simulink model "hpt_frt_model"  (R2025a)
settings: Solver=ode3  StartTime=0.0  StopTime=0.5  FixedStep=1e-05  RelTol=1e-3
undefined symbols (not defined in the file or in its folder): D1, Delta
libraries: spsSeriesRLCBranchLib x5, spsUniversalBridgeLib x4, spsLinearTransformerLib x3, spsThreePhaseFaultLib x2, spsThreePhaseVIMeasurementLib x2, spsBreakerLib x1, spsThreePhaseSourceLib x1, spsThreePhaseParallelRLCLoadLib x1, spsThreePhaseTransformerTwoWindingsLib x1, spsVoltageMeasurementLib x1, sps_lib x1
settings Model: Creator=m1391  LastModifiedBy=m1391

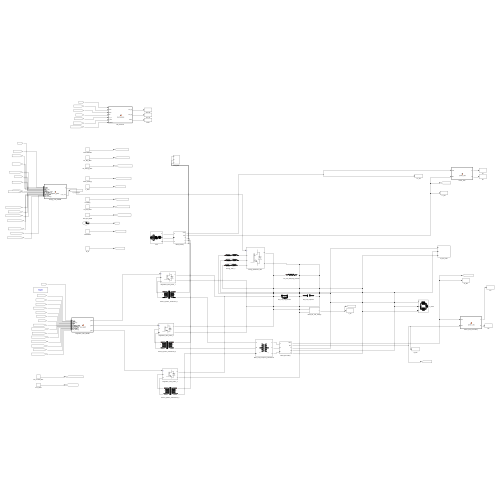
[thumbnail: Simulink's stored preview of the top-level diagram]
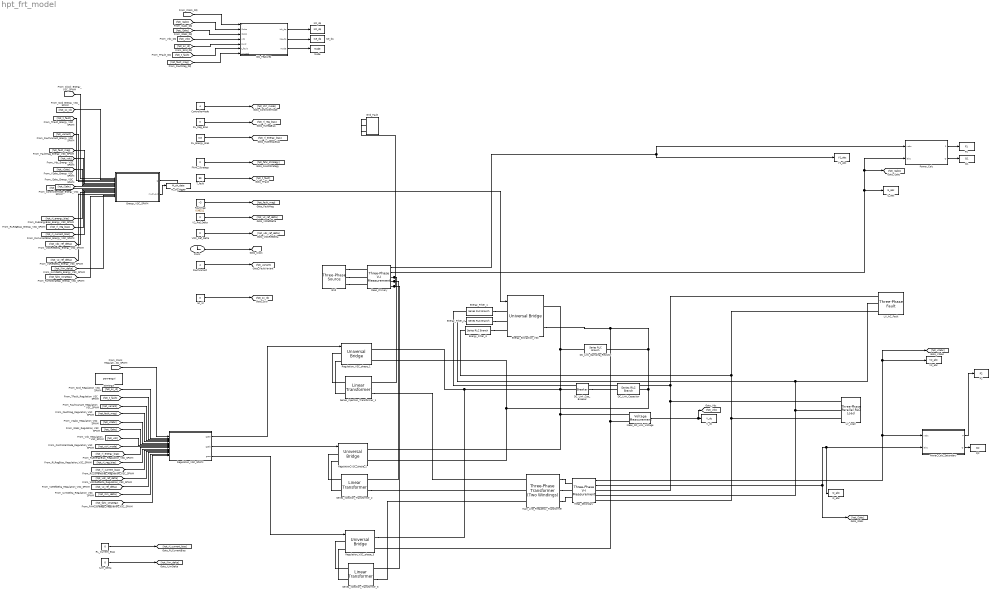
== system hpt_frt_model ==
  Clock : Clock
  ControllerMode : Constant  Value=4
  DC_Link_Cap_Breaker : spsBreakerLib/Breaker  InitialState=1  SwitchingTimes=[99]  External=off  BreakerResistance=0.01  SnubberResistance=1e6  SnubberCapacitance=inf  Measurements=None  MoreParameters=on  NoBreakLoop=off
  DC_Link_Capacitor : spsSeriesRLCBranchLib/Series RLC Branch  LConnTagsString=__new0  RConnTagsString=__new0  BranchType=C  Resistance=1  Inductance=1e-3  SetiL0=off  InitialCurrent=0  Capacitance=2200e-6  Setx0=on  InitialVoltage=800  Measurements=None
  DC_Link_Damping_Resistor : spsSeriesRLCBranchLib/Series RLC Branch  LConnTagsString=__new0  RConnTagsString=__new0  BranchType=R  Resistance=8.2  Inductance=1e-3  SetiL0=off  InitialCurrent=0  Capacitance=1e-6  Setx0=off  InitialVoltage=0  Measurements=None
  DQ_Features : MATLAB Function  TreatAsAtomicUnit=on
  Energy_Extraction_VSC : spsUniversalBridgeLib/Universal Bridge  Arms=3  SnubberResistance=1e5  SnubberCapacitance=1e-9  Device=IGBT / Diodes  Ron=1e-3  Lon=0  ForwardVoltages="[  0  0  ]"  ForwardVoltage=0  GTOparameters=[ 10e-6 , 20e-6 ]  IGBTparameters=[ 1e-6 , 2e-6 ]  Measurements=All voltages and currents  Measurements_2=None  converterType=Rectifier
  Energy_Filter_1 : spsSeriesRLCBranchLib/Series RLC Branch  LConnTagsString=__new0  RConnTagsString=__new0  BranchType=RL  Resistance=0.05  Inductance=0.003  SetiL0=off  InitialCurrent=0  Capacitance=1e-6  Setx0=off  InitialVoltage=0  Measurements=None
  Energy_Filter_2 : spsSeriesRLCBranchLib/Series RLC Branch  LConnTagsString=__new0  RConnTagsString=__new0  BranchType=RL  Resistance=0.05  Inductance=0.003  SetiL0=off  InitialCurrent=0  Capacitance=1e-6  Setx0=off  InitialVoltage=0  Measurements=None
  Energy_Filter_3 : spsSeriesRLCBranchLib/Series RLC Branch  LConnTagsString=__new0  RConnTagsString=__new0  BranchType=RL  Resistance=0.05  Inductance=0.003  SetiL0=off  InitialCurrent=0  Capacitance=1e-6  Setx0=off  InitialVoltage=0  Measurements=None
  Energy_VSC_SPWM : MATLAB Function  TreatAsAtomicUnit=on
  FAHC_Strategy : Constant  Value=0
  FaultMag : Constant  Value=0.98311
  FaultVariant : Constant  Value=4
  Grid : spsThreePhaseSourceLib/Three-Phase Source  InternalConnection=Yg  VoltagePhases=off  Voltage=10000  PhaseAngle=0  Voltage_phases=[25e3 25e3 25e3]/sqrt(3)  PhaseAngles_phases=[0 -120 +120]  Frequency=50  NonIdealSource=on  SpecifyImpedance=on  Resistance=0.1  Inductance=0.00095493  ShortCircuitLevel=100e6  BaseVoltage=25e3  XRratio=7  BusType=swing  Pref=10e3  Qref=0  Prefabc=[10e3, 10e3, 10e3]  Qrefabc=[0, 0, 0]  Qmin=-inf  Qmax=inf
  Grid_Fault : spsThreePhaseFaultLib/Three-Phase Fault  InitialStates=0  FaultA=on  FaultB=on  FaultC=on  GroundFault=on  SwitchTimes=[0.30 0.45]  External=off  SwitchStatus=NaN  FaultResistance=300  GroundResistance=0.001  SnubberResistance=1e6  SnubberCapacitance=inf  Measurements=None
  I1_abc : ToWorkspace  VariableName=I1_abc  SampleTime=5e-05
  I2_abc : ToWorkspace  VariableName=I2_abc  SampleTime=5e-05
  ILim_Delta : Constant  Value=0
  Ise_dq : ToWorkspace  VariableName=Ise_dq  SampleTime=5e-05
  Ish_dq : ToWorkspace  VariableName=Ish_dq  SampleTime=5e-05
  LV_AC_Fault : spsThreePhaseFaultLib/Three-Phase Fault  InitialStates=0  FaultA=off  FaultB=off  FaultC=off  GroundFault=off  SwitchTimes=[99 100]  External=off  SwitchStatus=NaN  FaultResistance=0.2977  GroundResistance=0.2977  SnubberResistance=1e6  SnubberCapacitance=inf  Measurements=None
  LV_Load : spsThreePhaseParallelRLCLoadLib/Three-Phase Parallel RLC Load  LConnTagsString=A|B|C  Configuration=Y (grounded)  NominalVoltage=400  Vabc=[1e3 1e3 1e3]  Vabcp=[1e3 1e3 1e3]  NominalFrequency=50  UnbalancedPower=off  ActivePower=281649.2048  InductivePower=143907.1654  CapacitivePower=0  Pabc=[10e3 9e3 11e3]  QLabc=[100 90 110]  QCabc=[100 90 110]  Pabcp=[10e3 9e3 11e3]  QLabcp=[100 90 110]  QCabcp=[100 90 110]  Measurements=None  LoadType=constant Z
  Main_Line_Frequency_Transformer : spsThreePhaseTransformerTwoWindingsLib/Three-Phase Transformer (Two Windings)  Winding1Connection=Delta (D1)  Winding2Connection=Yg  CoreType=Three single-phase transformers  SetSaturation=off  Hysteresis=off  DataFile='hysteresis'  SetInitialFlux=off  Measurements=None  UNITS=pu  NominalPower=[400000 50]  Winding1=[10000 0.002 0.01]  Winding2=[400 0.002 0.01]  Rm=500  Lm=500  L0=0.5  Saturation=[ 0,0 ; 0.0024,1.2 ; 1.0,1.52 ]  InitialFluxes=[ 0.8 , -0.8 , 0.7 ]  BreakLoop=off  DiscreteSolver=Trapezoidal iterative  DataType=off  TransfoNumber=1
  Meas_DC_Link_Voltage : spsVoltageMeasurementLib/Voltage Measurement  PhasorSimulation=off  OutputType=Magnitude  PSBequivalent=0
  Meas_Primary : spsThreePhaseVIMeasurementLib/Three-Phase V-I Measurement  VoltageMeasurement=phase-to-ground  SetLabelV=off  LabelV=Vabc  Vpu=off  VpuLL=off  CurrentMeasurement=yes  SetLabelI=off  LabelI=Iabc  Ipu=off  Pbase=100e6  Vbase=500e3  OutputType=Complex  PhasorSimulation=off  PSBequivalent=0
  Meas_Secondary : spsThreePhaseVIMeasurementLib/Three-Phase V-I Measurement  VoltageMeasurement=phase-to-ground  SetLabelV=off  LabelV=Vabc  Vpu=off  VpuLL=off  CurrentMeasurement=yes  SetLabelI=off  LabelI=Iabc  Ipu=off  Pbase=100e6  Vbase=500e3  OutputType=Complex  PhasorSimulation=off  PSBequivalent=0
  P1 : ToWorkspace  VariableName=P1  SampleTime=5e-05
  P2 : ToWorkspace  VariableName=P2  SampleTime=5e-05
  Power_Calc : MATLAB Function  TreatAsAtomicUnit=on
  Power_Calc_Secondary : MATLAB Function  TreatAsAtomicUnit=on
  Q1 : ToWorkspace  VariableName=Q1  SampleTime=5e-05
  Q2 : ToWorkspace  VariableName=Q2  SampleTime=5e-05
  RL_Current_Bias : Constant  Value=0
  RL_Energy_Bias : Constant  Value=0.8
  RL_Reg_Bias : Constant  Value=0
  Regulation_VSC_SPWM : MATLAB Function  TreatAsAtomicUnit=on
  Regulation_VSC_phase_1 : spsUniversalBridgeLib/Universal Bridge  Arms=2  SnubberResistance=1e5  SnubberCapacitance=1e-9  Device=IGBT / Diodes  Ron=1e-3  Lon=0  ForwardVoltages="[  0  0  ]"  ForwardVoltage=0  GTOparameters=[ 10e-6 , 20e-6 ]  IGBTparameters=[ 1e-6 , 2e-6 ]  Measurements=All voltages and currents  Measurements_2=None  converterType=Rectifier
  Regulation_VSC_phase_2 : spsUniversalBridgeLib/Universal Bridge  Arms=2  SnubberResistance=1e5  SnubberCapacitance=1e-9  Device=IGBT / Diodes  Ron=1e-3  Lon=0  ForwardVoltages="[  0  0  ]"  ForwardVoltage=0  GTOparameters=[ 10e-6 , 20e-6 ]  IGBTparameters=[ 1e-6 , 2e-6 ]  Measurements=All voltages and currents  Measurements_2=None  converterType=Rectifier
  Regulation_VSC_phase_3 : spsUniversalBridgeLib/Universal Bridge  Arms=2  SnubberResistance=1e5  SnubberCapacitance=1e-9  Device=IGBT / Diodes  Ron=1e-3  Lon=0  ForwardVoltages="[  0  0  ]"  ForwardVoltage=0  GTOparameters=[ 10e-6 , 20e-6 ]  IGBTparameters=[ 1e-6 , 2e-6 ]  Measurements=All voltages and currents  Measurements_2=None  converterType=Rectifier
  Sc_id : Constant  Value=0
  Series_Injection_Transformer_1 : spsLinearTransformerLib/Linear Transformer  UNITS=pu  NominalPower=[40000 50]  winding1=[400 0.001 0.001]  winding2=[1154.7005 0.001 0.001]  ThreeWindings=off  winding3=[ 315e3 0.002 0.08 ]  RmLm=[500 500]  Measurements=None  DataType=off
  Series_Injection_Transformer_2 : spsLinearTransformerLib/Linear Transformer  UNITS=pu  NominalPower=[40000 50]  winding1=[400 0.001 0.001]  winding2=[1154.7005 0.001 0.001]  ThreeWindings=off  winding3=[ 315e3 0.002 0.08 ]  RmLm=[500 500]  Measurements=None  DataType=off
  Series_Injection_Transformer_3 : spsLinearTransformerLib/Linear Transformer  UNITS=pu  NominalPower=[40000 50]  winding1=[400 0.001 0.001]  winding2=[1154.7005 0.001 0.001]  ThreeWindings=off  winding3=[ 315e3 0.002 0.08 ]  RmLm=[500 500]  Measurements=Winding voltages  DataType=off
  T_fault : Constant  Value=99
  V1_abc : ToWorkspace  VariableName=V1_abc  SampleTime=5e-05
  V2_Ref_Delta : Constant  Value=0
  V2_abc : ToWorkspace  VariableName=V2_abc  SampleTime=5e-05
  VDC_Ref_Delta : Constant  Value=0
  V_dc : ToWorkspace  VariableName=V_dc  SampleTime=5e-05
  m_sh_logger : ToWorkspace  VariableName=M_sh_data  SampleTime=-1
  mode : ToWorkspace  VariableName=mode  SampleTime=5e-05
  powergui : sps_lib/powergui  Priority=1  SimulationMode=Discrete  SampleTime=1e-05  frequency=60  Iterations=50  frequencyindice=50  Pbase=100e6  ErrMax=1e-4  UnitsV=kV  UnitsW=MW  buscounter=0  FunctionMessages=off  echomessages=off  EnableUseOfTLC=off  CurrentSourceSwitches=off  DisableSnubberDevices=off  DisableRonSwitches=off  DisableVfSwitches=off  DisplayEquations=off  AutomaticDiscreteSolvers=off  SolverType=Tustin/Backward Euler (TBE)  Interpol=off  ExternalGateDelay=off  methode=off  Ts=100  x0status=blocks  SPID=on  SwTol=0  HookPort=off  NonlinearTolerance=1e-4  nMaxIteration=100  ContinueOnMaxIteration=off  RestoreLinks=warning  ResistiveCurrentMeasurement=off  Frange=[0:2:500]  Ylog=off  Xlog=on  ShowGrid=off  save=off  variable=ZData  structure=0  ZoomFFT=off  StartTime=0.0  cycles=1  DisplayStyle=1  fundamental=60  FreqAxis=off  MaxFrequency=1000  frequencyindicesteady=1  RmsSteady=1  display=off
  wires:
  [hpt_clk] -> DQ_Features/1(t)
  VDC_Ref_Delta/1 -> [hpt_vdc_ref_delta]
  ILim_Delta/1 -> [hpt_ilim_delta]
  T_fault/1 -> [hpt_t_fault]
  ControllerMode/1 -> [hpt_ctrl_mode]
  [hpt_i1abc] -> DQ_Features/2(i1abc)
  [hpt_i2abc] -> DQ_Features/3(i2abc)
  [hpt_ctrl_mode] -> Energy_VSC_SPWM/9(controller_mode)
  [hpt_clk] -> Energy_VSC_SPWM/1(t)
  [hpt_v2_ref_delta] -> Regulation_VSC_SPWM/14(v2_ref_delta)
  [hpt_vdc_ref_delta] -> Regulation_VSC_SPWM/13(vdc_ref_delta)
  [hpt_rl_reg_bias] -> Regulation_VSC_SPWM/11(rl_reg_bias)
  [hpt_t_fault] -> DQ_Features/6(t_fault)
  [hpt_v2abc] -> Energy_VSC_SPWM/7(v2abc)
  DQ_Features/1(Ish_dq) -> Ish_dq/1
  [hpt_t_fault] -> Energy_VSC_SPWM/3(t_fault)
  [hpt_vdc] -> DQ_Features/4(vdc)
  [hpt_sc_id] -> DQ_Features/5(sc_id)
  [hpt_fault_mag] -> Regulation_VSC_SPWM/5(fault_mag)
  RL_Energy_Bias/1 -> [hpt_rl_energy_bias]
  FaultMag/1 -> [hpt_fault_mag]
  [hpt_fault_mag] -> DQ_Features/7(unused)
  [hpt_ilim_delta] -> Regulation_VSC_SPWM/15(ilim_delta)
  [hpt_rl_current_bias] -> Regulation_VSC_SPWM/12(rl_current_bias)
  RL_Reg_Bias/1 -> [hpt_rl_reg_bias]
  [hpt_rl_energy_bias] -> Regulation_VSC_SPWM/10(rl_energy_bias)
  [hpt_i2abc] -> Regulation_VSC_SPWM/7(i2abc)
  FAHC_Strategy/1 -> [hpt_fahc_strategy]
  V2_Ref_Delta/1 -> [hpt_v2_ref_delta]
  Clock/1 -> [hpt_clk]
  FaultVariant/1 -> [hpt_variant]
  Sc_id/1 -> [hpt_sc_id]
  DQ_Features/2(Ise_dq) -> Ise_dq/1
  [hpt_vdc] -> Energy_VSC_SPWM/6(vdc)
  [hpt_sc_id] -> Energy_VSC_SPWM/2(sc_id)
  [hpt_v2abc] -> Regulation_VSC_SPWM/6(v2abc)
  [hpt_t_fault] -> Regulation_VSC_SPWM/3(t_fault)
  [hpt_clk] -> Regulation_VSC_SPWM/1(t)
  [hpt_v2_ref_delta] -> Energy_VSC_SPWM/14(v2_ref_delta)
  [hpt_vdc_ref_delta] -> Energy_VSC_SPWM/13(vdc_ref_delta)
  [hpt_rl_reg_bias] -> Energy_VSC_SPWM/11(rl_reg_bias)
  DQ_Features/3(mode) -> mode/1
  [hpt_sc_id] -> Regulation_VSC_SPWM/2(sc_id)
  [hpt_variant] -> Regulation_VSC_SPWM/4(variant)
  [hpt_fault_mag] -> Energy_VSC_SPWM/5(fault_mag)
  [hpt_vdc] -> Regulation_VSC_SPWM/8(vdc)
  [hpt_ctrl_mode] -> Regulation_VSC_SPWM/9(controller_mode)
  [hpt_variant] -> Energy_VSC_SPWM/4(variant)
  [hpt_fahc_strategy] -> Regulation_VSC_SPWM/16(fahc_strategy)
  [hpt_ilim_delta] -> Energy_VSC_SPWM/15(ilim_delta)
  Regulation_VSC_SPWM/3(gsec) -> Regulation_VSC_phase_3/1
  [hpt_i2abc] -> Energy_VSC_SPWM/8(i2abc)
  [hpt_rl_current_bias] -> Energy_VSC_SPWM/12(rl_current_bias)
  [hpt_rl_energy_bias] -> Energy_VSC_SPWM/10(rl_energy_bias)
  RL_Current_Bias/1 -> [hpt_rl_current_bias]
  Regulation_VSC_SPWM/1(gsea) -> Regulation_VSC_phase_1/1
  Regulation_VSC_SPWM/2(gseb) -> Regulation_VSC_phase_2/1
  [hpt_fahc_strategy] -> Energy_VSC_SPWM/16(fahc_strategy)
  Energy_VSC_SPWM/1(g) -> Energy_Extraction_VSC/1
  Meas_Primary/1 -> Power_Calc/1(vabc), V1_abc/1
  Meas_Primary/2 -> Power_Calc/2(iabc), [hpt_i1abc], I1_abc/1
  Meas_DC_Link_Voltage/1 -> [hpt_vdc], V_dc/1
  Power_Calc/1(P) -> P1/1
  Power_Calc/2(Q) -> Q1/1
  Meas_Secondary/1 -> [hpt_v2abc], V2_abc/1, Power_Calc_Secondary/1(vabc)
  Meas_Secondary/2 -> Power_Calc_Secondary/2(iabc), I2_abc/1, [hpt_i2abc]
  Power_Calc_Secondary/1(P) -> P2/1
  Power_Calc_Secondary/2(Q) -> Q2/1
  Energy_VSC_SPWM/2(m_sh_out) -> m_sh_logger/1
  connections:
  Regulation_VSC_phase_3/LConn1 -- Series_Injection_Transformer_3/LConn1
  Regulation_VSC_phase_3/LConn2 -- Series_Injection_Transformer_3/LConn2
  Energy_Filter_1/LConn1 -- LV_AC_Fault/LConn1 -- Meas_Secondary/RConn1 -- LV_Load/LConn1
  Energy_Filter_2/LConn1 -- Meas_Secondary/RConn2 -- LV_Load/LConn2 -- LV_AC_Fault/LConn2
  Energy_Filter_3/LConn1 -- Meas_Secondary/RConn3 -- LV_Load/LConn3 -- LV_AC_Fault/LConn3
  Energy_Filter_1/RConn1 -- Energy_Extraction_VSC/LConn1
  Energy_Filter_2/RConn1 -- Energy_Extraction_VSC/LConn2
  Energy_Filter_3/RConn1 -- Energy_Extraction_VSC/LConn3
  Regulation_VSC_phase_3/RConn1 -- Energy_Extraction_VSC/RConn1 -- DC_Link_Damping_Resistor/LConn1 -- DC_Link_Cap_Breaker/LConn1 -- Regulation_VSC_phase_2/RConn1 -- Meas_DC_Link_Voltage/LConn1 -- Regulation_VSC_phase_1/RConn1
  Grid/RConn1 -- Meas_Primary/LConn1
  Grid/RConn2 -- Meas_Primary/LConn2
  Grid/RConn3 -- Meas_Primary/LConn3
  Energy_Extraction_VSC/RConn2 -- Regulation_VSC_phase_2/RConn2 -- Regulation_VSC_phase_1/RConn2 -- DC_Link_Capacitor/RConn1 -- DC_Link_Damping_Resistor/RConn1 -- Regulation_VSC_phase_3/RConn2 -- Meas_DC_Link_Voltage/LConn2
  DC_Link_Cap_Breaker/RConn1 -- DC_Link_Capacitor/LConn1
  Regulation_VSC_phase_1/LConn2 -- Series_Injection_Transformer_1/LConn2
  Regulation_VSC_phase_1/LConn1 -- Series_Injection_Transformer_1/LConn1
  Regulation_VSC_phase_2/LConn2 -- Series_Injection_Transformer_2/LConn2
  Regulation_VSC_phase_2/LConn1 -- Series_Injection_Transformer_2/LConn1
  Series_Injection_Transformer_1/RConn1 -- Meas_Primary/RConn1 -- Grid_Fault/LConn1
  Series_Injection_Transformer_2/RConn1 -- Meas_Primary/RConn2 -- Grid_Fault/LConn2
  Series_Injection_Transformer_3/RConn1 -- Meas_Primary/RConn3 -- Grid_Fault/LConn3
  Series_Injection_Transformer_1/RConn2 -- Main_Line_Frequency_Transformer/LConn1
  Series_Injection_Transformer_2/RConn2 -- Main_Line_Frequency_Transformer/LConn2
  Series_Injection_Transformer_3/RConn2 -- Main_Line_Frequency_Transformer/LConn3
  Main_Line_Frequency_Transformer/RConn1 -- Meas_Secondary/LConn1
  Main_Line_Frequency_Transformer/RConn2 -- Meas_Secondary/LConn2
  Main_Line_Frequency_Transformer/RConn3 -- Meas_Secondary/LConn3

== matlab function hpt_frt_model/Energy_VSC_SPWM ==
  data: t input; g output; sc_id input; t_fault input; variant input; fault_mag input; vdc input; v2abc input; i2abc input; controller_mode input; rl_energy_bias input; rl_reg_bias input; rl_current_bias input; vdc_ref_delta input; v2_ref_delta input; ilim_delta input; fahc_strategy input; m_sh_out output
function [g, m_sh_out] = spwm_gates(t,sc_id,t_fault,variant,fault_mag,vdc,v2abc,i2abc,controller_mode,rl_energy_bias,rl_reg_bias,rl_current_bias,vdc_ref_delta,v2_ref_delta,ilim_delta,fahc_strategy)
%#codegen
persistent ivdc last_t
if isempty(ivdc) || t < 1e-9
    ivdc = 0; last_t = t;
end
dt = max(0, min(1e-4, t - last_t));
last_t = t;
f1 = 50; fc = 5000;
theta = 2*pi*f1*t;
carrier = 2*abs(2*(fc*t - floor(fc*t + 0.5))) - 1;
v2 = real(v2abc);
i2 = real(i2abc);
vll = sqrt(((v2(1)-v2(2))^2 + (v2(2)-v2(3))^2 + (v2(3)-v2(1))^2)/3);
vpu = vll / 400;
ipu = max(abs(i2)) / 816.5;
if int32(controller_mode) == 7
    strat = int32(0);
    if t >= t_fault + 0.005; strat = int32(fahc_strategy); end
    if strat == 1; vdc_ref_eff = 760.0;
    elseif strat == 2; vdc_ref_eff = 740.0;
    elseif strat == 3; vdc_ref_eff = 720.0;
    else; vdc_ref_eff = 800.0; end
elseif int32(controller_mode) == 6
    vdc_ref_eff = max(720.0, min(840.0, 800.0 + vdc_ref_delta));
else
    vdc_ref_eff = 800.0;
end
evdc = (vdc_ref_eff - abs(vdc)) / vdc_ref_eff;
ivdc = min(0.35, max(-0.35, ivdc + evdc*dt*350));
m = 0.68 + 0.30*evdc + 0.08*ivdc;
if int32(controller_mode) == 3
    [m_ai, ~] = dnn_frt_policy(abs(vdc)/800, vpu, ipu, double(t >= t_fault), sc_id);
    m = m_ai;
end
if int32(sc_id) == 6 || int32(sc_id) == 7
    if t >= t_fault
        if int32(controller_mode) ~= 3 && int32(controller_mode) ~= 4 && int32(controller_mode) ~= 6 && int32(controller_mode) ~= 7
            m = min(m, 0.32);
        end
    end
end
if int32(controller_mode) == 4
    if t >= t_fault && (int32(sc_id) == 6 || int32(sc_id) == 7)
        m = min(m, 0.42);
    end
end
if int32(controller_mode) == 5
    e_bias = min(1.0, max(-1.0, rl_energy_bias));
    cur_bias = min(1.0, max(-1.0, rl_current_bias));
    m = m + 0.14*e_bias;
    if t >= t_fault && (int32(sc_id) == 6 || int32(sc_id) == 7)
        m = min(m, 0.42 + 0.16*max(0, e_bias));
    end
    if ipu > 2.0 + 0.8*max(0, cur_bias)
        m = min(m, 0.20 + 0.08*max(0, cur_bias));
    end
end
if int32(controller_mode) == 6 || int32(controller_mode) == 7
    if t >= t_fault && (int32(sc_id) == 6 || int32(sc_id) == 7)
        m = min(m, 0.42);
    end
end
% Mode 9: SAC direct modulation — branch-free
% rl_energy_bias interpreted as direct m_sh [0, 0.9]
% Pre-fault: nominal PI active; post-fault: SAC command
m9 = double(int32(controller_mode) == 9);
if_fault9 = double(t >= t_fault) * m9;
m_sh_cmd = max(0.0, min(0.90, rl_energy_bias));
m_pre9 = min(0.90, max(0.20, 0.68 + 0.30*evdc + 0.08*ivdc));
m = (1-m9)*m + m9*(if_fault9*m_sh_cmd + (1-if_fault9)*m_pre9);
% Protection floors anchored to 800V (LVRT criterion is absolute)
if abs(vdc) > 920.0 || ipu > 2.0
    m = min(m, 0.25);
end
if abs(vdc) > 1048.0 || ipu > 3.0
    m = min(m, 0.12);
end
if abs(vdc) < 780.0
    m = max(m, 0.64);
end
if abs(vdc) < 740.0
    m = max(m, 0.78);
end
if abs(vdc) < 700.0
    m = max(m, 0.86);
end
if abs(vdc) < 600.0
    m = max(m, 0.90);
end
m = min(0.92, max(0.20, m));
% ── Mode 10: voltage-mode STATCOM reactive support (FRT) ──
m10 = double(int32(controller_mode) == 10);
iq10 = max(-0.30, min(0.30, rl_current_bias));   % SAC reactive cmd i_sh_q (pu)
boost10 = m10 * double(t >= t_fault) * (0.9 * iq10);  % +cap raises VSC mag -> supports weak-grid PCC
if abs(vdc) > 1048.0; boost10 = min(boost10, 0.0); end  % do not add reactive if DC already over
m = min(0.95, max(0.05, m + boost10));
va = m*sin(theta);
vb = m*sin(theta - 2*pi/3);
vc = m*sin(theta + 2*pi/3);
ga = va >= carrier;
gb = vb >= carrier;
gc = vc >= carrier;
g = double([ga; ~ga; gb; ~gb; gc; ~gc]);
m_sh_out = m;   % expose shunt modulation index for measurement
if t >= t_fault && (int32(sc_id) == 3 || int32(sc_id) == 8)
    idx = max(1,min(6,int32(variant)));
    scale = max(0,min(1,1 - fault_mag));
    g(idx) = g(idx)*scale;
end

== matlab function hpt_frt_model/Regulation_VSC_SPWM ==
  data: t input; gsea output; sc_id input; t_fault input; variant input; fault_mag input; v2abc input; i2abc input; vdc input; controller_mode input; rl_energy_bias input; rl_reg_bias input; rl_current_bias input; vdc_ref_delta input; v2_ref_delta input; ilim_delta input; fahc_strategy input; gseb output; gsec output
function [gsea,gseb,gsec] = vse_spwm(t,sc_id,t_fault,variant,fault_mag,v2abc,i2abc,vdc,controller_mode,rl_energy_bias,rl_reg_bias,rl_current_bias,vdc_ref_delta,v2_ref_delta,ilim_delta,fahc_strategy)
%#codegen
persistent ivac last_t
if isempty(ivac) || t < 1e-9
    ivac = 0; last_t = t;
end
dt = max(0, min(1e-4, t - last_t));
last_t = t;
f1 = 50; fc = 5000;
theta = 2*pi*f1*t;
carrier = 2*abs(2*(fc*t - floor(fc*t + 0.5))) - 1;
v2 = real(v2abc);
i2 = real(i2abc);
vll = sqrt(((v2(1)-v2(2))^2 + (v2(2)-v2(3))^2 + (v2(3)-v2(1))^2)/3);
vpu = vll / 400;
ipu = max(abs(i2)) / 816.5;
sag = max(0, 0.98 - vpu);
m = min(0.24, max(0.02, 0.045 + 0.42*sag));
if int32(controller_mode) == 4
    ev = 1.0 - vpu;
    ivac = min(0.20, max(-0.20, ivac + ev*dt*80));
    m = 0.030 + 0.55*max(0, ev) + 0.18*ivac;
    if abs(vdc) < 720
        m = min(m, 0.06);
    end
    if abs(vdc) > 960
        m = min(m, 0.04);
    end
end
if int32(controller_mode) == 5
    ev = 1.0 - vpu;
    reg_bias = min(1.0, max(-1.0, rl_reg_bias));
    cur_bias = min(1.0, max(-1.0, rl_current_bias));
    ivac = min(0.24, max(-0.24, ivac + ev*dt*(80 + 40*max(0, reg_bias))));
    m = 0.030 + (0.55 + 0.20*reg_bias)*max(0, ev) + 0.18*ivac + 0.05*reg_bias;
    if abs(vdc) < 720
        m = min(m, 0.08 + 0.03*max(0, reg_bias));
    end
    if abs(vdc) > 960
        m = min(m, 0.04 + 0.02*max(0, cur_bias));
    end
end
if int32(controller_mode) == 3
    [~, m_ai] = dnn_frt_policy(abs(vdc)/800, vpu, ipu, double(t >= t_fault), sc_id);
    m = m_ai;
end
if int32(controller_mode) == 6 || int32(controller_mode) == 7
    if int32(controller_mode) == 7
        strat = int32(0);
        if t >= t_fault + 0.005; strat = int32(fahc_strategy); end
        if strat == 1; vdc_ref_eff = 760.0; ilim_eff = 2.8;
        elseif strat == 2; vdc_ref_eff = 740.0; ilim_eff = 2.8;
        elseif strat == 3; vdc_ref_eff = 720.0; ilim_eff = 2.5;
        else; vdc_ref_eff = 800.0; ilim_eff = 3.0; end
        v2_ref_eff = 400.0;
    else
        v2_ref_eff = 400.0;
        vdc_ref_eff = max(720.0, min(840.0, 800.0 + vdc_ref_delta));
        ilim_eff   = max(2.5,   min(3.5,   3.0   + ilim_delta));
    end
    ev = (v2_ref_eff / 400.0) - vpu;
    ivac = min(0.20, max(-0.20, ivac + ev*dt*80));
    m = 0.030 + 0.55*max(0, ev) + 0.18*ivac;
    if abs(vdc) < 720.0
        m = min(m, 0.06);
    end
    if abs(vdc) > 960.0
        m = min(m, 0.04);
    end
    if ipu > ilim_eff
        m = min(m, 0.02);
    end
end
if int32(sc_id) == 6 || int32(sc_id) == 7
    if t >= t_fault
        if int32(controller_mode) ~= 3 && int32(controller_mode) ~= 4 && int32(controller_mode) ~= 6 && int32(controller_mode) ~= 7
            m = 0.015;
        end
    end
end
ipu_limit = 2.0;
if int32(controller_mode) == 5
    ipu_limit = 2.0 + 0.8*max(0, min(1.0, rl_current_bias));
end
if ipu > ipu_limit && int32(controller_mode) ~= 6 && int32(controller_mode) ~= 7
    m = min(m, 0.02 + 0.04*max(0, min(1.0, rl_current_bias)));
end
% Mode 9: SAC direct series modulation
% Deep fault (V2<0.20 pu): fall back to Mode 4 PI + current limiter
% so the H-bridge is properly regulated during sc_3ph (not 50% duty)
phi9 = 0.0;
if int32(controller_mode) == 9
    if vpu >= 0.20
        m_se_d9 = max(-0.30, min(0.30, rl_reg_bias));
        m_se_q9 = max(-0.30, min(0.30, rl_current_bias));
        m = min(0.30, sqrt(m_se_d9^2 + m_se_q9^2 + 1e-12));
        phi9 = atan2(m_se_q9, m_se_d9 + 1e-9);
    else
        ev_d = max(0.0, 1.0 - vpu);
        m = 0.030 + 0.55*ev_d;
        if abs(vdc) < 720.0; m = min(m, 0.06); end
        if abs(vdc) > 960.0; m = min(m, 0.04); end
        if ipu > 2.0; m = min(m, 0.02); end
    end
end
m = min(0.30, max(0.0, m));
va_ref = m*sin(theta + phi9);
vb_ref = m*sin(theta - 2*pi/3 + phi9);
vc_ref = m*sin(theta + 2*pi/3 + phi9);
ga = va_ref >= carrier;
gb = vb_ref >= carrier;
gc = vc_ref >= carrier;
gsea = double([ga; ~ga; ~ga; ga]);
gseb = double([gb; ~gb; ~gb; gb]);
gsec = double([gc; ~gc; ~gc; gc]);
if t >= t_fault && (int32(sc_id) == 4 || int32(sc_id) == 8)
    idx = max(1,min(4,int32(variant)));
    scale = max(0,min(1,1 - fault_mag));
    if idx == 1, gsea(1) = gsea(1)*scale; end
    if idx == 2, gsea(2) = gsea(2)*scale; end
    if idx == 3, gsea(3) = gsea(3)*scale; end
    if idx == 4, gsea(4) = gsea(4)*scale; end
end

== matlab function hpt_frt_model/Power_Calc ==
  data: vabc input; P output; iabc input; Q output
function [P,Q] = power_calc(vabc,iabc)
%#codegen
P = sum(vabc .* iabc);
alpha_v = (2/3)*(vabc(1)-0.5*vabc(2)-0.5*vabc(3));
beta_v = (2/3)*(sqrt(3)/2)*(vabc(2)-vabc(3));
alpha_i = (2/3)*(iabc(1)-0.5*iabc(2)-0.5*iabc(3));
beta_i = (2/3)*(sqrt(3)/2)*(iabc(2)-iabc(3));
Q = 1.5*(beta_v*alpha_i - alpha_v*beta_i);

== matlab function hpt_frt_model/Power_Calc_Secondary ==
  data: vabc input; P output; iabc input; Q output
function [P,Q] = power_calc(vabc,iabc)
%#codegen
P = sum(vabc .* iabc);
alpha_v = (2/3)*(vabc(1)-0.5*vabc(2)-0.5*vabc(3));
beta_v = (2/3)*(sqrt(3)/2)*(vabc(2)-vabc(3));
alpha_i = (2/3)*(iabc(1)-0.5*iabc(2)-0.5*iabc(3));
beta_i = (2/3)*(sqrt(3)/2)*(iabc(2)-iabc(3));
Q = 1.5*(beta_v*alpha_i - alpha_v*beta_i);

== matlab function hpt_frt_model/DQ_Features ==
  data: t input; Ish_dq output; i1abc input; i2abc input; vdc input; sc_id input; t_fault input; unused input; Ise_dq output; mode output
function [Ish_dq,Ise_dq,mode] = dq_features(t,i1abc,i2abc,vdc,sc_id,t_fault,~)
%#codegen
% Ish_dq(1): dc_err_proxy = 0.05*(800-Vdc) + 0.02*(id1-id2)
% Ish_dq(2): Iq2_kA = iq2/1000 (secondary q-axis current, kA units)
theta = 2*pi*50*t;
c = [cos(theta); cos(theta-2*pi/3); cos(theta+2*pi/3)];
s = [-sin(theta); -sin(theta-2*pi/3); -sin(theta+2*pi/3)];
id2 = (2/3)*sum(i2abc .* c);
iq2 = (2/3)*sum(i2abc .* s);
id1 = (2/3)*sum(i1abc .* c);
iq1 = (2/3)*sum(i1abc .* s);
fault = double(t >= t_fault);
dc_sig = 0.05*(800-vdc) + 0.02*(id1-id2);
Ish_dq = [dc_sig; iq2/1000];
Ise_dq = [(id1-id2)/1000; (iq1-iq2)/1000];
mode = 1 + fault * double(sc_id > 0);
